simulink model "Walker_Delta"  (R2022b)
settings: Solver=FixedStepAuto  StartTime=0  StopTime=86400  FixedStep=SampleTime  RelTol=1e-3
model workspace (MAT data in the model file):
  SampleTime = 30
  Sim_Time = 31556952
  StartDate = [2024 4 16 0 0 0]
  StartTime = datetime
  StartTime.data = 1713225600000
  T_prog = 3180
  missionSatellites.SemiMajorAxis = [6871000; 6871000; 6871000; 6871000; 6871000; 6871000; 6871000; 6871000; 6871000; 6871000; 6871000; 6871000; 6871000; 6871000; 6871000; 6871000; 6871000; 6871000; 6871000; 6871000; 6871000; 6871000; 6871000; 6871000; 6871000; 6871000; 6871000; 6871000; 6871000; 6871000; 6871000; 6871000; 6871000; 6871000; 6871000; 6871000; 6871000; 6871000; 6871000; 6871000; 6871000; 6871000; 6871000; 6871000; 6871000; 6871000; 6871000; 6871000; 6871000; 6871000; 6871000; 6871000; 6871000; 6871000; 6871000; 6871000; 6871000; 6871000; 6871000; 6871000; 6871000; 6871000; 6871000; 6871000; 6871000; 6871000; 6871000; 6871000; 6871000; 6871000; 6871000; 6871000]
  missionSatellites.Eccentricity = [0; 0; 0; 0; 0; 0; 0; 0; 0; 0; 0; 0; 0; 0; 0; 0; 0; 0; 0; 0; 0; 0; 0; 0; 0; 0; 0; 0; 0; 0; 0; 0; 0; 0; 0; 0; 0; 0; 0; 0; 0; 0; 0; 0; 0; 0; 0; 0; 0; 0; 0; 0; 0; 0; 0; 0; 0; 0; 0; 0; 0; 0; 0; 0; 0; 0; 0; 0; 0; 0; 0; 0]
  missionSatellites.Inclination = [56; 56; 56; 56; 56; 56; 56; 56; 56; 56; 56; 56; 56; 56; 56; 56; 56; 56; 56; 56; 56; 56; 56; 56; 56; 56; 56; 56; 56; 56; 56; 56; 56; 56; 56; 56; 56; 56; 56; 56; 56; 56; 56; 56; 56; 56; 56; 56; 56; 56; 56; 56; 56; 56; 56; 56; 56; 56; 56; 56; 56; 56; 56; 56; 56; 56; 56; 56; 56; 56; 56; 56]
  missionSatellites.ArgOfPeriapsis = [0; 0; 0; 0; 0; 0; 0; 0; 0; 0; 0; 0; 0; 0; 0; 0; 0; 0; 0; 0; 0; 0; 0; 0; 0; 0; 0; 0; 0; 0; 0; 0; 0; 0; 0; 0; 0; 0; 0; 0; 0; 0; 0; 0; 0; 0; 0; 0; 0; 0; 0; 0; 0; 0; 0; 0; 0; 0; 0; 0; 0; 0; 0; 0; 0; 0; 0; 0; 0; 0; 0; 0]
  missionSatellites.RAAN = [0; 0; 0; 0; 0; 0; 0; 0; 0; 0; 0; 0; 0; 0; 0; 0; 0; 0; 0; 0; 0; 0; 0; 0; 120; 120; 120; 120; 120; 120; 120; 120; 120; 120; 120; 120; 120; 120; 120; 120; 120; 120; 120; 120; 120; 120; 120; 120; 240; 240; 240; 240; 240; 240; 240; 240; 240; 240; 240; 240; 240; 240; 240; 240; 240; 240; 240; 240; 240; 240; 240; 240]
  missionSatellites.TrueAnomaly = [0; 15; 30; 45; 60; 75; 90; 105; 120; 135; 150; 165; 180; 195; 210; 225; 240; 255; 270; 285; 300; 315; 330; 345; 5; 20; 35; 50; 65; 80; 95; 110; 125; 140; 155; 170; 185; 200; 215; 230; 245; 260; 275; 290; 305; 320; 335; 350; 10; 25; 40; 55; 70; 85; 100; 115; 130; 145; 160; 175; 190; 205; 220; 235; 250; 265; 280; 295; 310; 325; 340; 355]
  missionSatellites.ConstellationDefinition = table
  missionSatellites.ConstellationDefinition.data{1} = [6871000; 6871000; 6871000; 6871000; 6871000; 6871000; 6871000; 6871000; 6871000; 6871000; 6871000; 6871000; 6871000; 6871000; 6871000; 6871000; 6871000; 6871000; 6871000; 6871000; 6871000; 6871000; 6871000; 6871000; 6871000; 6871000; 6871000; 6871000; 6871000; 6871000; 6871000; 6871000; 6871000; 6871000; 6871000; 6871000; 6871000; 6871000; 6871000; 6871000; 6871000; 6871000; 6871000; 6871000; 6871000; 6871000; 6871000; 6871000; 6871000; 6871000; 6871000; 6871000; 6871000; 6871000; 6871000; 6871000; 6871000; 6871000; 6871000; 6871000; 6871000; 6871000; 6871000; 6871000; 6871000; 6871000; 6871000; 6871000; 6871000; 6871000; 6871000; 6871000]
  missionSatellites.ConstellationDefinition.data{2} = [0; 0; 0; 0; 0; 0; 0; 0; 0; 0; 0; 0; 0; 0; 0; 0; 0; 0; 0; 0; 0; 0; 0; 0; 0; 0; 0; 0; 0; 0; 0; 0; 0; 0; 0; 0; 0; 0; 0; 0; 0; 0; 0; 0; 0; 0; 0; 0; 0; 0; 0; 0; 0; 0; 0; 0; 0; 0; 0; 0; 0; 0; 0; 0; 0; 0; 0; 0; 0; 0; 0; 0]
  missionSatellites.ConstellationDefinition.data{3} = [56; 56; 56; 56; 56; 56; 56; 56; 56; 56; 56; 56; 56; 56; 56; 56; 56; 56; 56; 56; 56; 56; 56; 56; 56; 56; 56; 56; 56; 56; 56; 56; 56; 56; 56; 56; 56; 56; 56; 56; 56; 56; 56; 56; 56; 56; 56; 56; 56; 56; 56; 56; 56; 56; 56; 56; 56; 56; 56; 56; 56; 56; 56; 56; 56; 56; 56; 56; 56; 56; 56; 56]
  missionSatellites.ConstellationDefinition.data{4} = [0; 0; 0; 0; 0; 0; 0; 0; 0; 0; 0; 0; 0; 0; 0; 0; 0; 0; 0; 0; 0; 0; 0; 0; 120; 120; 120; 120; 120; 120; 120; 120; 120; 120; 120; 120; 120; 120; 120; 120; 120; 120; 120; 120; 120; 120; 120; 120; 240; 240; 240; 240; 240; 240; 240; 240; 240; 240; 240; 240; 240; 240; 240; 240; 240; 240; 240; 240; 240; 240; 240; 240]
  missionSatellites.ConstellationDefinition.data{5} = [0; 0; 0; 0; 0; 0; 0; 0; 0; 0; 0; 0; 0; 0; 0; 0; 0; 0; 0; 0; 0; 0; 0; 0; 0; 0; 0; 0; 0; 0; 0; 0; 0; 0; 0; 0; 0; 0; 0; 0; 0; 0; 0; 0; 0; 0; 0; 0; 0; 0; 0; 0; 0; 0; 0; 0; 0; 0; 0; 0; 0; 0; 0; 0; 0; 0; 0; 0; 0; 0; 0; 0]
  missionSatellites.ConstellationDefinition.data{6} = [0; 15; 30; 45; 60; 75; 90; 105; 120; 135; 150; 165; 180; 195; 210; 225; 240; 255; 270; 285; 300; 315; 330; 345; 5; 20; 35; 50; 65; 80; 95; 110; 125; 140; 155; 170; 185; 200; 215; 230; 245; 260; 275; 290; 305; 320; 335; 350; 10; 25; 40; 55; 70; 85; 100; 115; 130; 145; 160; 175; 190; 205; 220; 235; 250; 265; 280; 295; 310; 325; 340; 355]
  missionSatellites.ConstellationDefinition.ndims = 2
  missionSatellites.ConstellationDefinition.nrows = 72
  missionSatellites.ConstellationDefinition.nvars = 6
  missionSatellites.ConstellationDefinition.varnames = {'a_m_', 'e', 'i_deg_', 'x__deg_', 'x__deg__1', 'x__deg__2'}
  missionSatellites.ConstellationDefinition.props.useVariableNamesOriginal = 1
  missionSatellites.ConstellationDefinition.props.useDimensionNamesOriginal = 0
  missionSatellites.ConstellationDefinition.props.CustomProps = struct()
  missionSatellites.ConstellationDefinition.props.VariableCustomProps = struct()
  missionSatellites.ConstellationDefinition.props.versionSavedFrom = 4
  missionSatellites.ConstellationDefinition.props.minCompatibleVersion = 1
  missionSatellites.ConstellationDefinition.props.incompatibilityMsg = ''
  missionSatellites.ConstellationDefinition.props.VersionSavedFrom = 4
  missionSatellites.ConstellationDefinition.props.Description = ''
  missionSatellites.ConstellationDefinition.props.VariableNamesOriginal = {'a (m)', 'e', 'i (deg)', 'Ω (deg)', 'ω (deg)', 'θ (deg)'}
  missionSatellites.ConstellationDefinition.props.DimensionNames = {'Row', 'Variables'}
  missionSatellites.ConstellationDefinition.props.DimensionNamesOriginal = {}
  missionSatellites.ConstellationDefinition.props.UserData = []
  missionSatellites.ConstellationDefinition.props.VariableDescriptions = {}
  missionSatellites.ConstellationDefinition.props.VariableUnits = {}
  missionSatellites.ConstellationDefinition.props.VariableContinuity = {}
  r = [0 0 0]
  v = [0 0 0]
values from neighbouring files (symbols this model uses):
  StartTime = datetime(StartDate)    [TLEsearch_tool.m]
undefined symbols (not defined in the file or in its folder): cputime, datevec
libraries: matrix_library x3, simulink x2
settings Model: PauseTimes=60  Creator=Matteo  LastModifiedBy=Matteo
settings DataIOCC: SignalLogging=off  DSMLogging=off  OutputSaveName=LLA  DatasetSignalFormat=timetable  LoggingFileName=LLA.mat

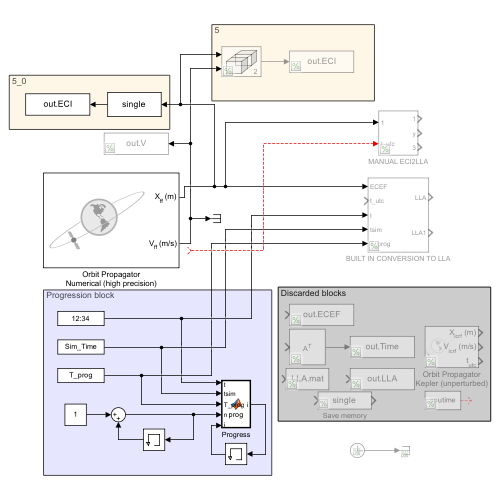
[thumbnail: Simulink's stored preview of the top-level diagram]
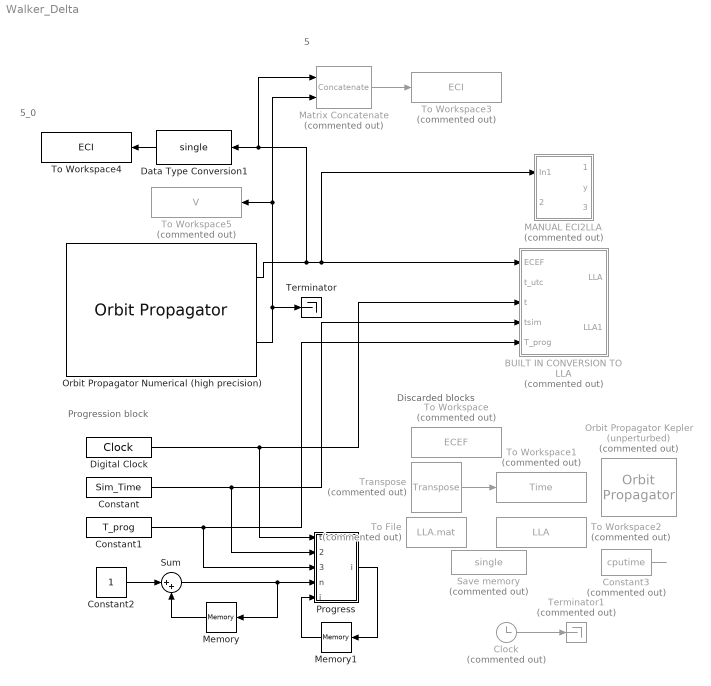
== system Walker_Delta ==
  note: 5_0
  note: 5
  note: Discarded blocks
  note: Progression block
  BUILT IN CONVERSION TO LLA : Subsystem  Commented=on
  Clock : Clock  Commented=on
  Constant : Constant  Value=Sim_Time
  Constant1 : Constant  Value=T_prog
  Constant2 : Constant
  Constant3 : Constant  Commented=on  Value=cputime
  Data Type Conversion1 : DataTypeConversion  OutDataTypeStr=single  RndMeth=Round  SaturateOnIntegerOverflow=off
  Digital Clock : DigitalClock  SampleTime=T_prog
  MANUAL ECI2LLA : Subsystem  Commented=on
  Matrix Concatenate : Concatenate  Commented=on  Mode=Multidimensional array  ConcatenateDimension=2
  Memory : Memory
  Memory1 : Memory
  Orbit Propagator Kepler (unperturbed) : OrbitPropagator  Commented=on  startDate=datevec(StartTime)  stateFormatKep=ICRF state vector  inertialPosition=r  inertialVelocity=v  fixedPosition=[-4142689.0 -2676864.7 -4669861.6]  fixedVelocity=[1452.7 -6720.7 2568.1]  customR=3396200  customMu=4.305e13  customJ2=1.0826269e-03  customOmega=4.06125949e-3  timeFormat=Gregorian
  Orbit Propagator Numerical (high precision) : OrbitPropagator  propagator=Numerical (high precision)  outportFrame=Fixed-frame  startDate=StartDate  dateOut=off  action=None  semiMajorAxis=missionSatellites.SemiMajorAxis  eccentricity=missionSatellites.Eccentricity  inclination=missionSatellites.Inclination  raan=missionSatellites.RAAN  argPeriapsis=missionSatellites.ArgOfPeriapsis  trueAnomaly=missionSatellites.TrueAnomaly  inertialPosition=[0,0,0]  inertialVelocity=[0,0,0]  fixedPosition=[0,0,0]  fixedVelocity=[0,0,0]  gravityModel=Point-mass  customR=3396200  customMu=4.305e13  customJ2=1.0826269e-03  customOmega=4.06125949e-3  useEOPs=off  timeFormat=Gregorian
  Progress : MATLAB Function  TreatAsAtomicUnit=on
  Save memory : DataTypeConversion  Commented=on  OutDataTypeStr=single  RndMeth=Round  SaturateOnIntegerOverflow=off
  Sum : Sum  Inputs=|++
  Terminator : Terminator
  Terminator1 : Terminator  Commented=on
  To File : ToFile  Commented=on  Filename=LLA.mat  MatrixName=LLA  SaveFormat=Timeseries
  To Workspace : ToWorkspace  Commented=on  VariableName=ECEF  SampleTime=-1
  To Workspace1 : ToWorkspace  Commented=on  VariableName=Time  SampleTime=-1
      settings: Save2DSignal=2-D array (concatenate along first dimension)
  To Workspace2 : ToWorkspace  Commented=on  VariableName=LLA  SampleTime=-1
  To Workspace3 : ToWorkspace  Commented=on  VariableName=ECI  SampleTime=-1
  To Workspace4 : ToWorkspace  VariableName=ECI  SampleTime=-1
  To Workspace5 : ToWorkspace  Commented=on  VariableName=V  SaveFormat=Timeseries  SampleTime=-1
  Transpose : matrix_library/Transpose  Commented=on
  wires:
  Transpose/1 -> To Workspace1/1
  Digital Clock/1 -> BUILT IN CONVERSION TO LLA/3(t), Progress/1(t)
  Constant1/1 -> BUILT IN CONVERSION TO LLA/5(T_prog), Progress/3(T_prog)
  Constant/1 -> BUILT IN CONVERSION TO LLA/4(tsim), Progress/2(tsim)
  Orbit Propagator Numerical (high precision)/1 -> BUILT IN CONVERSION TO LLA/1(ECEF), MANUAL ECI2LLA/1(In1), Data Type Conversion1/1, Matrix Concatenate/1
  Constant2/1 -> Sum/1
  Sum/1 -> Memory/1, Progress/4(n)
  Memory/1 -> Sum/2
  Progress/1(i) -> Memory1/1
  Memory1/1 -> Progress/5("i ")
  Constant3/1 -> ?
  Orbit Propagator Numerical (high precision)/2 -> Terminator/1, Matrix Concatenate/2, To Workspace5/1
  ? -> MANUAL ECI2LLA/2(t_utc)
  Data Type Conversion1/1 -> To Workspace4/1
  Clock/1 -> Terminator1/1
  Matrix Concatenate/1 -> To Workspace3/1

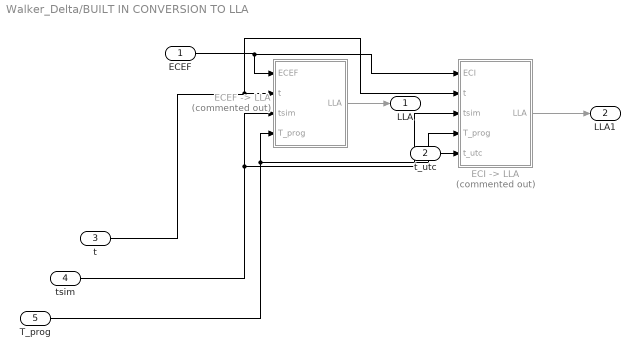
== system Walker_Delta/BUILT IN CONVERSION TO LLA ==
  ECEF : Inport
  t_utc : Inport  Port=2
  t : Inport  Port=3
  tsim : Inport  Port=4
  T_prog : Inport  Port=5
  "ECEF -> LLA" : MATLAB Function  Commented=on  TreatAsAtomicUnit=on
  "ECI -> LLA" : MATLAB Function  Commented=on  TreatAsAtomicUnit=on
  LLA : Outport
  LLA1 : Outport  Port=2
  wires:
  tsim/1 -> "ECEF -> LLA"/3(tsim), "ECI -> LLA"/3(tsim)
  ECEF/1 -> "ECI -> LLA"/1(ECI), "ECEF -> LLA"/1(ECEF)
  t/1 -> "ECI -> LLA"/2(t), "ECEF -> LLA"/2(t)
  t_utc/1 -> "ECI -> LLA"/5(t_utc)
  T_prog/1 -> "ECEF -> LLA"/4(T_prog), "ECI -> LLA"/4(T_prog)
  "ECEF -> LLA"/1(LLA) -> LLA/1
  "ECI -> LLA"/1(LLA) -> LLA1/1

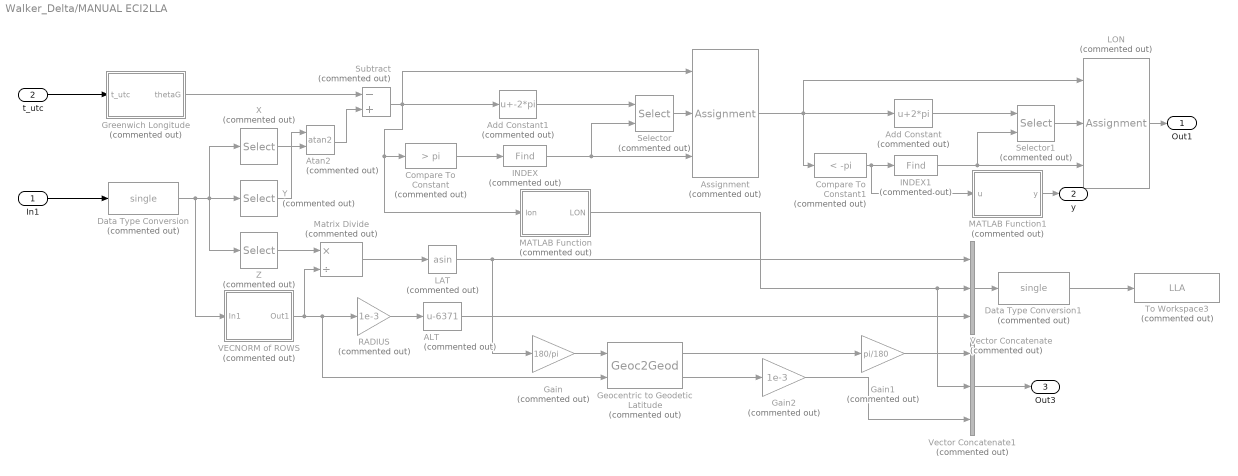
== system Walker_Delta/MANUAL ECI2LLA ==
  In1 : Inport
  t_utc : Inport  Port=2
  ALT : Bias  Commented=on  Bias=-6371  SaturateOnIntegerOverflow=off
  Add Constant : Bias  Commented=on  Bias=2*pi  SaturateOnIntegerOverflow=off
  Add Constant1 : Bias  Commented=on  Bias=-2*pi  SaturateOnIntegerOverflow=off
  Assignment : Assignment  Commented=on  DiagnosticForDimensions=Warning  IndexOptions=Index vector (port)  Indices=1  OutputSizes=1  RuntimeRangeChecks=on
  Atan2 : Trigonometry  Commented=on  Operator=atan2
  Compare To Constant : simulink/Logic and Bit Operations/Compare To Constant  Commented=on  relop=>  const=pi  OutDataTypeStr=boolean
  Compare To Constant1 : simulink/Logic and Bit Operations/Compare To Constant  Commented=on  relop=<  const=-pi  OutDataTypeStr=boolean
  Data Type Conversion : DataTypeConversion  Commented=on  OutDataTypeStr=single  RndMeth=Round  SaturateOnIntegerOverflow=off
  Data Type Conversion1 : DataTypeConversion  Commented=on  OutDataTypeStr=single  SaturateOnIntegerOverflow=off  RndMeth=Floor
  Gain : Gain  Commented=on  Gain=180/pi
  Gain1 : Gain  Commented=on  Gain=pi/180
  Gain2 : Gain  Commented=on  Gain=1e-3
  Geocentric to Geodetic Latitude : Geoc2Geod  Commented=on  outputAltitude=on
  Greenwich Longitude : MATLAB Function  Commented=on  TreatAsAtomicUnit=on
  INDEX : Find  Commented=on  NumberOfInputDimensions=1
  INDEX1 : Find  Commented=on  NumberOfInputDimensions=1
  LAT : Trigonometry  Commented=on  Operator=asin
  LON : Assignment  Commented=on  DiagnosticForDimensions=Warning  IndexOptions=Index vector (port)  Indices=1  OutputSizes=1  RuntimeRangeChecks=on
  MATLAB Function : MATLAB Function  Commented=on  TreatAsAtomicUnit=on
  MATLAB Function1 : MATLAB Function  Commented=on  TreatAsAtomicUnit=on
  Matrix Divide : Product  Commented=on  Inputs=*/
  RADIUS : Gain  Commented=on  Gain=1e-3
  Selector : Selector  Commented=on  IndexOptions=Index vector (port)  Indices=[1 3]  OutputSizes=1  RuntimeRangeChecks=on
  Selector1 : Selector  Commented=on  IndexOptions=Index vector (port)  Indices=[1 3]  OutputSizes=1  RuntimeRangeChecks=on
  Subtract : Sum  Commented=on  Inputs=-+
  To Workspace3 : ToWorkspace  Commented=on  VariableName=LLA  SaveFormat=Timeseries  SampleTime=-1
  VECNORM of ROWS : Subsystem  Commented=on
  Vector Concatenate : Concatenate  Commented=on  NumInputs=3  Mode=Multidimensional array  ConcatenateDimension=2
  Vector Concatenate1 : Concatenate  Commented=on  NumInputs=3  Mode=Multidimensional array  ConcatenateDimension=2
  X : Selector  Commented=on  NumberOfDimensions=2  InputPortWidth=3  IndexOptions=Select all,Index vector (dialog)  Indices=[1 3],1  OutputSizes=1,1  RuntimeRangeChecks=on
  Y : Selector  Commented=on  NumberOfDimensions=2  InputPortWidth=3  IndexOptions=Select all,Index vector (dialog)  Indices=[1 3],2  OutputSizes=1,1  RuntimeRangeChecks=on
  Z : Selector  Commented=on  NumberOfDimensions=2  InputPortWidth=3  IndexOptions=Select all,Index vector (dialog)  Indices=[1 3],3  OutputSizes=1,1  RuntimeRangeChecks=on
  Out1 : Outport
  y : Outport  Port=2
  Out3 : Outport  Port=3
  wires:
  Data Type Conversion1/1 -> To Workspace3/1
  VECNORM of ROWS/1(Out1) -> Matrix Divide/2, RADIUS/1, Geocentric to Geodetic Latitude/2
  Y/1 -> Atan2/1
  Add Constant/1 -> Selector1/1
  Geocentric to Geodetic Latitude/2 -> Gain2/1
  Data Type Conversion/1 -> VECNORM of ROWS/1(In1), Z/1, X/1, Y/1
  X/1 -> Atan2/2
  LON/1 -> Out1/1
  Compare To Constant1/1 -> INDEX1/1, MATLAB Function1/1(u)
  MATLAB Function/1(LON) -> Vector Concatenate/2, Vector Concatenate1/2
  INDEX1/1 -> LON/3, Selector1/2
  Matrix Divide/1 -> LAT/1
  Geocentric to Geodetic Latitude/1 -> Gain1/1
  Assignment/1 -> Compare To Constant1/1, Add Constant/1, LON/1
  MATLAB Function1/1(y) -> y/1
  Greenwich Longitude/1(thetaG) -> Subtract/1
  Subtract/1 -> MATLAB Function/1(lon), Compare To Constant/1, Add Constant1/1, Assignment/1
  Z/1 -> Matrix Divide/1
  t_utc/1 -> Greenwich Longitude/1(t_utc)
  Selector1/1 -> LON/2
  Gain/1 -> Geocentric to Geodetic Latitude/1
  Selector/1 -> Assignment/2
  Vector Concatenate1/1 -> Out3/1
  Compare To Constant/1 -> INDEX/1
  Gain1/1 -> Vector Concatenate1/1
  Gain2/1 -> Vector Concatenate1/3
  LAT/1 -> Gain/1, Vector Concatenate/1
  RADIUS/1 -> ALT/1
  ALT/1 -> Vector Concatenate/3
  Add Constant1/1 -> Selector/1
  Atan2/1 -> Subtract/2
  In1/1 -> Data Type Conversion/1
  Vector Concatenate/1 -> Data Type Conversion1/1
  INDEX/1 -> Assignment/3, Selector/2

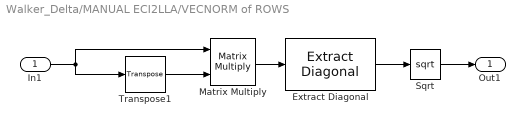
== system Walker_Delta/MANUAL ECI2LLA/VECNORM of ROWS ==
  In1 : Inport
  Extract Diagonal : matrix_library/Extract Diagonal
      settings: LibrarySourceBlock=|
      | simulink/Matrix
      | Operations/Extract Diagonal
  Matrix Multiply : Product  Multiplication=Matrix(*)
  Sqrt : Sqrt
  Transpose1 : matrix_library/Transpose
  Out1 : Outport
  wires:
  Sqrt/1 -> Out1/1
  Transpose1/1 -> Matrix Multiply/2
  Matrix Multiply/1 -> Extract Diagonal/1
  In1/1 -> Transpose1/1, Matrix Multiply/1
  Extract Diagonal/1 -> Sqrt/1

== matlab function Walker_Delta/BUILT IN CONVERSION TO LLA/ECI -> LLA ==
  data: LLA output; ECI input; t input; tsim input; T_prog input; t_utc input
function LLA = postproc(ECI,t,tsim,T_prog,t_utc)
coder.extrinsic('eci2lla','fprintf')

% fprintf('\n%.0f %.0f; %.0f %.0f\n',size(ECI),size(t_utc'))
sz = size(ECI,2);
if sz == 1
    LLA = single(zeros(size(ECI'))); % Define the output type for the extrinsic call.
    LLA = single(eci2lla(ECI',t_utc')); % [deg,deg, m]
    
%     fprintf('\nyoo\n')
else
    sz = size(ECI,1);
    t_UTC = zeros(sz,6);
    t_UTC = repmat(t_utc',sz,1);
    LLA = single(zeros(size(ECI))); % Define the output type for the extrinsic call.
    LLA = single(eci2lla(ECI,t_UTC)); % [deg,deg, m]
end
LLA = [LLA(:,1:2)*pi/180,LLA(:,3)*1e-3];  % [rad,rad,km]

persistent firstTime

if isempty(firstTime)
    firstTime = false;
    fprintf(' Simulation progress:         ')
end

prog = 100*t/tsim;

% fprintf('\b\b\b\b\b%4.0f%%',prog)
fprintf('\b\b\b\b\b\b\b\b%7.3f%%',prog)

% T_prog = ceil(tsim/(100*30))*30; % check progress sample time
if tsim - t < T_prog
    fprintf('\b\b\b\b\b\b\b\b100.000%%')
end

== matlab function Walker_Delta/Progress ==
  data: t input; tsim input; T_prog input; n input; i input; i output
function i = prog(t,tsim,T_prog,n,i)
coder.extrinsic('fprintf')

persistent firstTime

if isempty(firstTime)
    firstTime = false;
    fprintf(' Simulation progress:         ')
end

prog = 100*t/tsim;

if i == 0 || abs(i - n) > T_prog
    i = n;
    fprintf('\b\b\b\b\b\b\b\b%7.3f%%',prog)
end

if tsim - t < T_prog
    fprintf('\b\b\b\b\b\b\b\b%7.3f%%',100)
end

end

== matlab function Walker_Delta/BUILT IN CONVERSION TO LLA/ECEF -> LLA ==
  data: LLA output; ECEF input; t input; tsim input; T_prog input
function LLA = postproc(ECEF,t,tsim,T_prog)
coder.extrinsic('ecef2lla','fprintf')

sz = size(ECEF,2);
if sz == 1
    LLA = single(zeros(size(ECEF'))); % Define the output type for the extrinsic call.
    LLA = single(ecef2lla(ECEF','wgs84')); % [deg,deg, m]
    
else
    LLA = single(zeros(size(ECEF))); % Define the output type for the extrinsic call.
    LLA = single(ecef2lla(ECEF,'wgs84')); % [deg,deg, m]
end
LLA = [LLA(:,1:2)*pi/180,LLA(:,3)*1e-3];  % [rad,rad,km]

persistent firstTime

if isempty(firstTime)
    firstTime = false;
    fprintf(' Simulation progress:         ')
end

prog = 100*t/tsim;

% fprintf('\b\b\b\b\b%4.0f%%',prog)
fprintf('\b\b\b\b\b\b\b\b%7.3f%%',prog)

% T_prog = ceil(tsim/(100*30))*30; % check progress sample time
if tsim - t < T_prog
    fprintf('\b\b\b\b\b\b\b\b100.000%%')
end

== matlab function Walker_Delta/MANUAL ECI2LLA/Greenwich Longitude ==
  data: t_utc input; thetaG output
function thetaG = LongG(t_utc)
% Long Greenwhich at t0
% INPUT:
%   t_utc0 : 1x6 initial time vector [YY,MM,DD,hh,mm,ss]
% OUTPUT:
%   tG0    : scalar, [rad]  

J0 = 367*t_utc(1)-fix(7/4*(t_utc(1)+fix((t_utc(2)+9)/12)))+fix(275/9*t_utc(2))+t_utc(3)+1721013.5;
T0 = (J0-2451545)/36525;
lonG0 = mod(100.4606184 + 36000.77004 * T0 + 0.000387933 * T0^2 - 2.583e-8 * T0^3,360); % [deg]
lonG  = mod(lonG0 + 360.98564724 * (t_utc(4) + t_utc(5)/60 + t_utc(6)/3600)/24,360); % [deg]
thetaG = lonG * pi/180; % [rad]

end

== matlab function Walker_Delta/MANUAL ECI2LLA/MATLAB Function ==
  data: lon input; LON output
function LON = FIND(lon)

I = find(lon > pi);
lon(I)  = lon(I) - 2*pi;

I = find(lon < -pi);
lon(I)  = lon(I) + 2*pi;

LON = lon;

end

== matlab function Walker_Delta/MANUAL ECI2LLA/MATLAB Function1 ==
  data: u input; y output
function y = FIND(u)

y = find(u);

end
